simulink library "Generator_Lib"  (R2019a)
settings: Solver=VariableStepAuto  StartTime=0.0  StopTime=10.0  RelTol=1e-3
undefined symbols (not defined in the file): block_angle, D1, Delta, DiscIntNeverNeededParam, fao, Ts
libraries: powerlib x56, powerlib_extras x9, simulink x8, sps_avr x2, powerlib_meascontrol x2
(part 1 of 2)
settings Model: Creator=smiller  LastModifiedBy=smiller

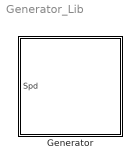
== system Generator_Lib ==
  Generator : Subsystem  VariantControlMode=Label  Variant=on  LabelModeActiveChoice=VSCF_DC_Link  mask{GenType=VSCF DC Link, GenTypeDCLink=Ideal}
      mask prompts: GenType "Generator Type"; GenTypeDCLink "Generator Type, DC Link"
      mask init:
      | set_param(gcb,'LabelModeActiveChoice',strrep(get_param(gcb,'GenType'),' ','_'));
      | set_param([gcb '/VSCF DC Link'],'GenTypeDCLink',get_param(gcb,'GenTypeDCLink'));
      settings: AttributesFormatString=%<BlockChoice>
      mask TypeOptions GenType: Ideal | Integrated Drive | VSCF Cycloconverter | VSCF DC Link
      mask TypeOptions GenTypeDCLink: Ideal | Sync Mach
      mask Display:
      | blk=find_system(gcbh, 'SearchDepth', 1,'FollowLinks','on','LookUnderMasks','all', 'Parent', gcb,'VariantObject', get_param(gcb,'activevariant'));
      | eval(get_param(blk, 'MaskDisplay'));

== system Generator_Lib/Generator ==
  Spd : Inport
  Ideal : Subsystem  VariantControl=Ideal
      mask Display: image(imread('Gen_Ideal_IMAGE.jpg'));
  Integrated Drive : Subsystem  VariantControl=Integrated_Drive
      mask Display: image(imread('Gen_IDG_IMAGE.jpg'))
  VSCF Cycloconverter : Subsystem  VariantControl=VSCF_Cycloconverter
      mask Display: image(imread('Gen_VSCF_Cycloconverter_IMAGE.jpg'))
  VSCF DC Link : Subsystem  VariantControl=VSCF_DC_Link  mask{GenTypeDCLink=Ideal}
      mask prompts: GenTypeDCLink "Generator Type"
      mask init:
      | set_param([gcb '/DC Link Gen'],'GenTypeDCLink',get_param(gcb,'GenTypeDCLink'));
      mask TypeOptions GenTypeDCLink: Ideal | Sync Mach
      mask Display: image('Gen_VSCF_DCLink_IMAGE.jpg');
  A : PMIOPort  Side=Right
  B : PMIOPort  Port=2  Side=Right
  C : PMIOPort  Port=3  Side=Right

== system Generator_Lib/Generator/Ideal ==
  Spd : Inport
  Parasitic Resistive Load : powerlib/Elements/Three-Phase Series RLC Load  LConnTagsString=A|B|C  Configuration=Y (grounded)  NominalVoltage=200  Vabc=[1e3 1e3 1e3]  Vabcp=[1e3 1e3 1e3]  NominalFrequency=400  UnbalancedPower=off  ActivePower=5000  InductivePower=0  CapacitivePower=0  Pabc=[10e3 9e3 11e3]  QLabc=[100 90 110]  QCabc=[100 90 110]  Pabcp=[10e3 9e3 11e3]  QLabcp=[100 90 110]  QCabcp=[100 90 110]  Measurements=None  LoadType=constant Z
      settings: SourceProductName=Simscape Electrical
  Sensing : Subsystem
      mask Display: disp('S')
  Terminator : Terminator
  Three-Phase V-I Measurement4 : powerlib/Measurements/Three-Phase V-I Measurement  VoltageMeasurement=phase-to-ground  SetLabelV=on  LabelV=Vabc_Gen1Only  Vpu=off  VpuLL=off  CurrentMeasurement=yes  SetLabelI=on  LabelI=Iabc_Gen1Only  Ipu=off  Pbase=100e6  Vbase=500e3  OutputType=Magnitude  PhasorSimulation=on  PSBequivalent=0
      settings: SourceProductName=Simscape Electrical
  Three-Phase Source : powerlib/Electrical Sources/Three-Phase Source  InternalConnection=Yg  VoltagePhases=off  Voltage=200  PhaseAngle=0  Voltage_phases=[25e3 25e3 25e3]/sqrt(3)  PhaseAngles_phases=[0 -120 +120]  Frequency=400  NonIdealSource=on  SpecifyImpedance=off  Resistance=0.1*0  Inductance=0.01*0  ShortCircuitLevel=0.1  BaseVoltage=200  XRratio=7  BusType=swing  Pref=0  Qref=0  Prefabc=[10e3, 10e3, 10e3]  Qrefabc=[0, 0, 0]  Qmin=-inf  Qmax=inf
      settings: SourceProductName=Simscape Electrical
  Vab : Subsystem
  rpm2 radps : Gain  Gain=pi/30
  A : PMIOPort  Side=Right
  B : PMIOPort  Port=2  Side=Right
  C : PMIOPort  Port=3  Side=Right
  wires:
  rpm2 radps/1 -> Terminator/1
  Spd/1 -> rpm2 radps/1
  connections:
  Three-Phase V-I Measurement4/LConn3 -- Three-Phase Source/RConn3
  Three-Phase V-I Measurement4/LConn2 -- Three-Phase Source/RConn2
  Three-Phase V-I Measurement4/LConn1 -- Three-Phase Source/RConn1
  A/RConn1 -- Parasitic Resistive Load/LConn1 -- Three-Phase V-I Measurement4/RConn1 -- Vab/RConn1
  C/RConn1 -- Three-Phase V-I Measurement4/RConn3 -- Parasitic Resistive Load/LConn3
  B/RConn1 -- Parasitic Resistive Load/LConn2 -- Three-Phase V-I Measurement4/RConn2 -- Vab/RConn2

== system Generator_Lib/Generator/Integrated Drive ==
  Spd : Inport
  Bus Selector2 : BusSelector  OutputSignals=Rotor speed wm (rad/s)
  Displays : Subsystem
  Generator Control Unit (GCU) : Subsystem
      mask Display: %image(imread('power_aircraft_distribution_GCU.jpg','jpg'))
  Generator Control Breaker (GCB) : Subsystem
  IDG : Subsystem
  Parasitic Resistive Load : powerlib/Elements/Three-Phase Series RLC Load  LConnTagsString=A|B|C  Configuration=Y (grounded)  NominalVoltage=200  Vabc=[1e3 1e3 1e3]  Vabcp=[1e3 1e3 1e3]  NominalFrequency=400  UnbalancedPower=off  ActivePower=5000  InductivePower=0  CapacitivePower=0  Pabc=[10e3 9e3 11e3]  QLabc=[100 90 110]  QCabc=[100 90 110]  Pabcp=[10e3 9e3 11e3]  QLabcp=[100 90 110]  QCabcp=[100 90 110]  Measurements=None  LoadType=constant Z
      settings: SourceProductName=Simscape Electrical
  Sensing : Subsystem
      mask Display: disp('S')
  Simplified Synchronous Machine SI Units : powerlib/Machines/Simplified Synchronous Machine SI Units  ConnectionType=3-wire Y  MechanicalLoad=Speed w  MeasurementBus=off  NominalParameters=[50e3 200 400]  Mechanical=[0.02 0 2]  InternalRL="[0.0204  0.08104e-3]"  InitialConditions=[-99 1.73677 24.5109 24.5109 24.5109 -1.98949 -121.989 118.011]  Units=1  LoadFlowParameters=[1 0 0 0 0]  TsPowergui=0  TsBlock=-1  BusType=swing  Pref=0  Qref=0  Qmin=-inf  Qmax=+inf  PLF=0  QLF=0
      settings: SourceProductName=Simscape Electrical  SourceProductBaseCode=PS
  Vab : Subsystem
  A : PMIOPort  Side=Right
  B : PMIOPort  Port=2  Side=Right
  C : PMIOPort  Port=3  Side=Right
  wires:
  IDG/1(Dr) -> Simplified Synchronous Machine SI Units/1
  Spd/1 -> IDG/1(Tur)
  Generator Control Breaker (GCB)/2(Iabc) -> Generator Control Unit (GCU)/1(Iabc)
  Generator Control Unit (GCU)/1(V Field) -> Simplified Synchronous Machine SI Units/2  "Field"
  Bus Selector2/1 -> Displays/1(w), Generator Control Unit (GCU)/3(PMG), Generator Control Breaker (GCB)/1(GLC)  "<Rotor speed wm (rad/s)>"
  Generator Control Breaker (GCB)/1(Vabc) -> Generator Control Unit (GCU)/2(Vabc)
  Simplified Synchronous Machine SI Units/1 -> Bus Selector2/1, Sensing/1(In1)
  connections:
  Simplified Synchronous Machine SI Units/RConn1 -- Generator Control Breaker (GCB)/LConn1 -- Parasitic Resistive Load/LConn1
  Simplified Synchronous Machine SI Units/RConn2 -- Generator Control Breaker (GCB)/LConn2 -- Parasitic Resistive Load/LConn2
  Simplified Synchronous Machine SI Units/RConn3 -- Parasitic Resistive Load/LConn3 -- Generator Control Breaker (GCB)/LConn3
  Generator Control Breaker (GCB)/RConn2 -- Vab/RConn2 -- B/RConn1
  C/RConn1 -- Generator Control Breaker (GCB)/RConn3
  Generator Control Breaker (GCB)/RConn1 -- Vab/RConn1 -- A/RConn1

== system Generator_Lib/Generator/VSCF Cycloconverter ==
  Spd : Inport
  AC Generator Cycloconverter : Subsystem
  Constant : Constant  Value=[0 0 0]
  Generator Control Breaker (GCB) : Subsystem
  Terminator : Terminator
  Terminator1 : Terminator
  Vab : Subsystem
  A : PMIOPort  Side=Right
  B : PMIOPort  Port=2  Side=Right
  C : PMIOPort  Port=3  Side=Right
  tag scope: Gen1Bus=global
  wires:
  Generator Control Breaker (GCB)/2(Iabc) -> Terminator1/1
  Generator Control Breaker (GCB)/1(Vabc) -> Terminator/1
  Constant/1 -> [Gen1Bus]
  Spd/1 -> Generator Control Breaker (GCB)/1(GLC), AC Generator Cycloconverter/1(rpm)
  connections:
  AC Generator Cycloconverter/RConn1 -- Generator Control Breaker (GCB)/LConn1
  AC Generator Cycloconverter/RConn2 -- Generator Control Breaker (GCB)/LConn2
  AC Generator Cycloconverter/RConn3 -- Generator Control Breaker (GCB)/LConn3
  B/RConn1 -- Generator Control Breaker (GCB)/RConn2 -- Vab/RConn2
  C/RConn1 -- Generator Control Breaker (GCB)/RConn3
  A/RConn1 -- Generator Control Breaker (GCB)/RConn1 -- Vab/RConn1

== system Generator_Lib/Generator/VSCF DC Link ==
  note: AC-DC-AC PWM Converter
  Spd : Inport
  Constant : Constant  Value=[0 0 0]
  DC Link Gen : Subsystem  VariantControlMode=Label  Variant=on  LabelModeActiveChoice=Ideal  mask{GenTypeDCLink=Ideal}
      mask prompts: GenTypeDCLink "Generator Type, DC Link"
      mask init:
      | set_param(gcb,'LabelModeActiveChoice',strrep(get_param(gcb,'GenTypeDCLink'),' ','_'));
      settings: AttributesFormatString=%<BlockChoice>
      mask TypeOptions GenTypeDCLink: Ideal | Sync Mach
  LC Filter : Subsystem
  Meas : powerlib/Measurements/Three-Phase V-I Measurement  VoltageMeasurement=phase-to-ground  SetLabelV=off  LabelV=V1  Vpu=on  VpuLL=off  CurrentMeasurement=no  SetLabelI=off  LabelI=I1  Ipu=off  Pbase=1e3  Vbase=200  OutputType=Magnitude  PhasorSimulation=off  PSBequivalent=0
      settings: SourceProductName=Simscape Electrical
  Rect and Inv : Subsystem
  Regulator : Subsystem
  Subsystem2 : Subsystem
      mask Display: disp('S')
  Subsystem4 : Subsystem
      mask Display: disp('S')
  Subsystem5 : Subsystem
      mask Display: disp('S')
  Transformer : powerlib/Elements/Three-Phase Transformer (Two Windings)  Winding1Connection=Yg  Winding2Connection=Delta (D1)  CoreType=Three single-phase transformers  SetSaturation=off  Hysteresis=off  DataFile='hysteresis'  SetInitialFlux=off  Measurements=None  UNITS=pu  NominalPower=[ 50e3 , 800 ]  Winding1=[ 200 , 0.004 , 0.02 ]  Winding2=[ 600 , 0.004 , 0.02 ]  Rm=200  Lm=200  L0=0.5  Saturation="[ 0,0  ;  0.005,1.2  ;  1.0,1.4 ]"  InitialFluxes=[ 0.8 , -0.8 , 0.7 ]  BreakLoop=off  DiscreteSolver=Trapezoidal iterative  DataType=off  TransfoNumber=0
      settings: SourceProductName=Simscape Electrical
  "Vref (pu) " : Constant
  A : PMIOPort  Side=Right
  B : PMIOPort  Port=2  Side=Right
  C : PMIOPort  Port=3  Side=Right
  tag scope: Gen1Bus=global
  wires:
  Constant/1 -> [Gen1Bus]
  Spd/1 -> DC Link Gen/1(rpm)
  Regulator/1(g) -> Rect and Inv/1(g)
  Meas/1 -> Regulator/2(Vabc (pu))
  "Vref (pu) "/1 -> Regulator/1(Vref (pu))
  connections:
  Rect and Inv/RConn3 -- LC Filter/LConn3
  Transformer/RConn3 -- Rect and Inv/LConn3
  Rect and Inv/LConn2 -- Transformer/RConn2
  DC Link Gen/RConn3 -- Transformer/LConn3
  Transformer/RConn1 -- Rect and Inv/LConn1
  Meas/LConn3 -- LC Filter/RConn3
  Meas/RConn3 -- C/RConn1
  Meas/LConn2 -- LC Filter/RConn2
  DC Link Gen/RConn2 -- Transformer/LConn2
  Meas/LConn1 -- LC Filter/RConn1
  B/RConn1 -- Meas/RConn2
  Rect and Inv/RConn1 -- Subsystem5/LConn1 -- LC Filter/LConn1
  Subsystem5/LConn2 -- Rect and Inv/RConn2 -- LC Filter/LConn2
  Subsystem2/LConn1 -- DC Link Gen/RConn1 -- Transformer/LConn1
  Meas/RConn1 -- A/RConn1 -- Subsystem4/LConn1

== system Generator_Lib/Generator/Ideal/Sensing ==
  Constant : Constant  Value=[1 1]*12000  SampleTime=-1
  Constant1 : Constant  Value=202  SampleTime=-1
  Mux : Mux  Inputs=3
  rpm2pu1 : Gain  Gain=2*pi/60
  tag scope: Gen1Data=global
  wires:
  Constant/1 -> rpm2pu1/1  "Spd"
  Mux/1 -> [Gen1Data]
  rpm2pu1/1 -> Mux/1
  Constant1/1 -> Mux/2
  [Pwr_Gen1_Only] -> Mux/3

== system Generator_Lib/Generator/Ideal/Vab ==
  Voltage Measurement : powerlib/Measurements/Voltage Measurement  PhasorSimulation=off  OutputType=Magnitude  PSBequivalent=0
      settings: SourceProductName=Simscape Electrical
  + : PMIOPort  Side=Right
  - : PMIOPort  Port=2  Side=Right
  tag scope: Gen1_Vab=global
  wires:
  Voltage Measurement/1 -> [Gen1_Vab]
  connections:
  Voltage Measurement/LConn2 -- -/RConn1
  Voltage Measurement/LConn1 -- +/RConn1

== system Generator_Lib/Generator/Integrated Drive/Displays ==
  w : Inport
  Frequency (Hz) : Display
      settings: Decimation=100  SampleTime=1e-2
  Gain : Gain  Gain=30/pi
  Gain3 : Gain  Gain=1/30
  Rate Transition : RateTransition  OutPortSampleTimeOpt=Inherit  OutPortSampleTime=Ts
  Rate Transition1 : RateTransition  OutPortSampleTimeOpt=Inherit  OutPortSampleTime=Ts
  Speed (RPM) : Display
      settings: Decimation=100  SampleTime=1e-2
  wires:
  Rate Transition1/1 -> Frequency (Hz)/1
  Gain/1 -> Gain3/1, Rate Transition/1
  Gain3/1 -> Rate Transition1/1
  Rate Transition/1 -> Speed (RPM)/1
  w/1 -> Gain/1

== system Generator_Lib/Generator/Integrated Drive/Generator Control Unit (GCU) ==
  Iabc : Inport
  Vabc : Inport  Port=2
  PMG : Inport  Port=3
  Demux : Demux  Outputs=3
  Excitation System : sps_avr/Excitation System  tr=20e-3  reg=[ 300, 0.001 ]  exc=[ 1, 0 ]  tgr=[ 0, 0 ]  damp=[ 0.001, 0.1 ]  sat=[ 0, 0 ]  lim=[ -2, 2, 0 ]  v0=[1 1*203.1/200]
      settings: SourceProductName=Simscape Electrical  SourceProductBaseCode=PS
  Integrator : Integrator
  PU_SI : Gain  Gain=200
  SI_PU : Gain  Gain=1/(200*sqrt(2))
  Terminator1 : Terminator
  Terminator2 : Terminator
  Vref : Constant
  abc to dq0 : powerlib_meascontrol/Transformations/abc to dq0  Alignment=90 degrees behind phase A axis
      settings: SourceProductName=Simscape Electrical
  threshold3 : Constant  Value=0
  V Field : Outport
  tag scope: Gen1_Vfield=global
  wires:
  Demux/3 -> Terminator2/1
  Iabc/1 -> Terminator1/1
  threshold3/1 -> Excitation System/4
  Vref/1 -> Excitation System/1
  PU_SI/1 -> [Gen1_Vfield], V Field/1
  Excitation System/1 -> PU_SI/1
  SI_PU/1 -> abc to dq0/1
  Demux/2 -> Excitation System/3
  Demux/1 -> Excitation System/2
  abc to dq0/1 -> Demux/1
  Integrator/1 -> abc to dq0/2
  PMG/1 -> Integrator/1
  Vabc/1 -> SI_PU/1

== system Generator_Lib/Generator/Integrated Drive/Generator Control Breaker (GCB) ==
  GLC : Inport
  Close switch : Subsystem
  Complex to Real-Imag : ComplexToRealImag  Output=Real
  Complex to Real-Imag1 : ComplexToRealImag  Output=Real
  Contactor : Subsystem
  Memory : Memory
  P.O.R  and CTA : powerlib/Measurements/Three-Phase V-I Measurement  VoltageMeasurement=phase-to-phase  SetLabelV=off  LabelV=Vabc_Gen1  Vpu=off  VpuLL=off  CurrentMeasurement=yes  SetLabelI=off  LabelI=Iabc_Gen1  Ipu=off  Pbase=100e6  Vbase=500e3  OutputType=Complex  PhasorSimulation=off  PSBequivalent=0
      settings: SourceProductName=Simscape Electrical
  in_a : PMIOPort  Side=Left
  in_b : PMIOPort  Port=2  Side=Left
  in_c : PMIOPort  Port=3  Side=Left
  out_a : PMIOPort  Port=4  Side=Right
  out_b : PMIOPort  Port=5  Side=Right
  out_c : PMIOPort  Port=6  Side=Right
  Vabc : Outport
  Iabc : Outport  Port=2
  wires:
  GLC/1 -> Memory/1
  P.O.R  and CTA/1 -> Complex to Real-Imag/1
  P.O.R  and CTA/2 -> Complex to Real-Imag1/1
  Complex to Real-Imag/1 -> Vabc/1
  Complex to Real-Imag1/1 -> Iabc/1
  Memory/1 -> Close switch/1(In1)
  Close switch/1(Out1) -> Contactor/1(com)
  connections:
  out_b/RConn1 -- Contactor/RConn2
  Contactor/LConn1 -- P.O.R  and CTA/RConn1
  P.O.R  and CTA/LConn1 -- in_a/RConn1
  in_b/RConn1 -- P.O.R  and CTA/LConn2
  P.O.R  and CTA/LConn3 -- in_c/RConn1
  Contactor/LConn3 -- P.O.R  and CTA/RConn3
  P.O.R  and CTA/RConn2 -- Contactor/LConn2
  Contactor/RConn1 -- out_a/RConn1
  Contactor/RConn3 -- out_c/RConn1

== system Generator_Lib/Generator/Integrated Drive/IDG ==
  Tur : Inport
  Constant : Constant  Value=12000*pi/30
  Terminator : Terminator
  rpm2 radps : Gain  Gain=pi/30
  Dr : Outport
  wires:
  Constant/1 -> Dr/1
  Tur/1 -> rpm2 radps/1
  rpm2 radps/1 -> Terminator/1

== system Generator_Lib/Generator/Integrated Drive/Sensing ==
  In1 : Inport
  Data : Subsystem
  Mux : Mux  Inputs=3
  tag scope: Gen1Data=global
  wires:
  Data/3(Pe) -> Mux/3
  Data/2(Vf) -> Mux/2
  Data/1(w) -> Mux/1
  In1/1 -> Data/1(B)
  Mux/1 -> [Gen1Data]

== system Generator_Lib/Generator/Integrated Drive/Vab ==
  Voltage Measurement : powerlib/Measurements/Voltage Measurement  PhasorSimulation=off  OutputType=Magnitude  PSBequivalent=0
      settings: SourceProductName=Simscape Electrical
  + : PMIOPort  Side=Right
  - : PMIOPort  Port=2  Side=Right
  tag scope: Gen1_Vab=global
  wires:
  Voltage Measurement/1 -> [Gen1_Vab]
  connections:
  Voltage Measurement/LConn1 -- +/RConn1
  Voltage Measurement/LConn2 -- -/RConn1

== system Generator_Lib/Generator/VSCF Cycloconverter/AC Generator Cycloconverter ==
  rpm : Inport
  Cycloconverter control (Vsync) : Subsystem
  Ground1 : powerlib/Elements/Ground  LConnTagsString=a
      settings: SourceProductName=Simscape Electrical
  Ideal Source : Subsystem
  Load Measurements : powerlib/Measurements/Three-Phase V-I Measurement  VoltageMeasurement=phase-to-ground  SetLabelV=on  LabelV=Vload  Vpu=off  VpuLL=off  CurrentMeasurement=yes  SetLabelI=on  LabelI=Iload  Ipu=off  Pbase=100e6  Vbase=500e3  OutputType=Complex  PhasorSimulation=off  PSBequivalent=0
      settings: SourceProductName=Simscape Electrical
  Phase A Cycloconverter : Subsystem
  Phase B Cycloconverter : Subsystem
  Phase C Cycloconverter : Subsystem
  Source Measurements : powerlib/Measurements/Three-Phase V-I Measurement  VoltageMeasurement=phase-to-ground  SetLabelV=on  LabelV=Vsource  Vpu=off  VpuLL=off  CurrentMeasurement=yes  SetLabelI=on  LabelI=Isource  Ipu=off  Pbase=100e6  Vbase=500e3  OutputType=Complex  PhasorSimulation=off  PSBequivalent=0
      settings: SourceProductName=Simscape Electrical
  Three-Phase Transformer (Two Windings)1 : powerlib/Elements/Three-Phase Transformer (Two Windings)  Winding1Connection=Delta (D1)  Winding2Connection=Delta (D1)  CoreType=Three single-phase transformers  SetSaturation=off  Hysteresis=off  DataFile='hysteresis'  SetInitialFlux=off  Measurements=None  UNITS=pu  NominalPower=[3e6 3000]  Winding1=[200 0 0]  Winding2=[200/sqrt(3) 1e-8 0]  Rm=Inf  Lm=Inf  L0=0.5  Saturation=[ 0,0 ; 0.0024,1.2 ; 1.0,1.52 ]  InitialFluxes=[ 0.8 , -0.8 , 0.7 ]  BreakLoop=off  DiscreteSolver=Trapezoidal iterative  DataType=off  TransfoNumber=1
      settings: SourceProductName=Simscape Electrical
  Three-Phase Transformer (Two Windings)2 : powerlib/Elements/Three-Phase Transformer (Two Windings)  Winding1Connection=Delta (D1)  Winding2Connection=Delta (D1)  CoreType=Three single-phase transformers  SetSaturation=off  Hysteresis=off  DataFile='hysteresis'  SetInitialFlux=off  Measurements=None  UNITS=pu  NominalPower=[3e6 3000]  Winding1=[200 0 0]  Winding2=[200/sqrt(3) 1e-8 0]  Rm=Inf  Lm=Inf  L0=0.5  Saturation=[ 0,0 ; 0.0024,1.2 ; 1.0,1.52 ]  InitialFluxes=[ 0.8 , -0.8 , 0.7 ]  BreakLoop=off  DiscreteSolver=Trapezoidal iterative  DataType=off  TransfoNumber=1
      settings: SourceProductName=Simscape Electrical
  Three-Phase Transformer (Two Windings)3 : powerlib/Elements/Three-Phase Transformer (Two Windings)  Winding1Connection=Delta (D1)  Winding2Connection=Delta (D1)  CoreType=Three single-phase transformers  SetSaturation=off  Hysteresis=off  DataFile='hysteresis'  SetInitialFlux=off  Measurements=None  UNITS=pu  NominalPower=[3e6 3000]  Winding1=[200 0 0]  Winding2=[200/sqrt(3) 1e-8 0]  Rm=Inf  Lm=Inf  L0=0.5  Saturation=[ 0,0 ; 0.0024,1.2 ; 1.0,1.52 ]  InitialFluxes=[ 0.8 , -0.8 , 0.7 ]  BreakLoop=off  DiscreteSolver=Trapezoidal iterative  DataType=off  TransfoNumber=1
      settings: SourceProductName=Simscape Electrical
  Vsync Measurement : powerlib/Measurements/Three-Phase V-I Measurement  VoltageMeasurement=phase-to-phase  SetLabelV=on  LabelV=Vsync  Vpu=off  VpuLL=off  CurrentMeasurement=no  SetLabelI=off  LabelI=Iabc  Ipu=off  Pbase=100e6  Vbase=500e3  OutputType=Complex  PhasorSimulation=off  PSBequivalent=0
      settings: SourceProductName=Simscape Electrical
  A : PMIOPort  Side=Right
  B : PMIOPort  Port=2  Side=Right
  C : PMIOPort  Port=3  Side=Right
  wires:
  rpm/1 -> Ideal Source/1(rpm)
  connections:
  Three-Phase Transformer (Two Windings)1/RConn3 -- Phase B Cycloconverter/LConn3
  Ideal Source/RConn3 -- Source Measurements/LConn3
  Load Measurements/RConn2 -- B/RConn1
  Ideal Source/RConn1 -- Source Measurements/LConn1
  Three-Phase Transformer (Two Windings)3/RConn2 -- Vsync Measurement/LConn2
  Source Measurements/LConn2 -- Ideal Source/RConn2
  Phase C Cycloconverter/LConn3 -- Three-Phase Transformer (Two Windings)2/RConn3
  Load Measurements/RConn3 -- C/RConn1
  Vsync Measurement/RConn3 -- Phase A Cycloconverter/LConn3
  Phase C Cycloconverter/RConn1 -- Load Measurements/LConn3
  Three-Phase Transformer (Two Windings)1/LConn2 -- Three-Phase Transformer (Two Windings)2/LConn2 -- Three-Phase Transformer (Two Windings)3/LConn2 -- Source Measurements/RConn2
  Three-Phase Transformer (Two Windings)1/LConn1 -- Three-Phase Transformer (Two Windings)2/LConn1 -- Three-Phase Transformer (Two Windings)3/LConn1 -- Source Measurements/RConn1
  Phase A Cycloconverter/RConn1 -- Load Measurements/LConn1
  Phase C Cycloconverter/LConn1 -- Three-Phase Transformer (Two Windings)2/RConn1
  Three-Phase Transformer (Two Windings)3/RConn1 -- Vsync Measurement/LConn1
  Phase B Cycloconverter/LConn2 -- Three-Phase Transformer (Two Windings)1/RConn2
  Phase B Cycloconverter/LConn1 -- Three-Phase Transformer (Two Windings)1/RConn1
  Vsync Measurement/RConn1 -- Phase A Cycloconverter/LConn1
  Phase B Cycloconverter/RConn1 -- Load Measurements/LConn2
  Three-Phase Transformer (Two Windings)1/LConn3 -- Source Measurements/RConn3 -- Three-Phase Transformer (Two Windings)3/LConn3 -- Three-Phase Transformer (Two Windings)2/LConn3
  Three-Phase Transformer (Two Windings)2/RConn2 -- Phase C Cycloconverter/LConn2
  Ground1/LConn1 -- Phase B Cycloconverter/RConn2 -- Phase A Cycloconverter/RConn2 -- Phase C Cycloconverter/RConn2
  Three-Phase Transformer (Two Windings)3/RConn3 -- Vsync Measurement/LConn3
  Phase A Cycloconverter/LConn2 -- Vsync Measurement/RConn2
  Load Measurements/RConn1 -- A/RConn1

== system Generator_Lib/Generator/VSCF Cycloconverter/Generator Control Breaker (GCB) ==
  GLC : Inport
  Close switch : Subsystem
  Complex to Real-Imag : ComplexToRealImag  Output=Real
  Complex to Real-Imag1 : ComplexToRealImag  Output=Real
  Contactor : Subsystem
  Memory : Memory
  P.O.R  and CTA : powerlib/Measurements/Three-Phase V-I Measurement  VoltageMeasurement=phase-to-phase  SetLabelV=off  LabelV=Vabc_Gen1  Vpu=off  VpuLL=off  CurrentMeasurement=yes  SetLabelI=off  LabelI=Iabc_Gen1  Ipu=off  Pbase=100e6  Vbase=500e3  OutputType=Complex  PhasorSimulation=off  PSBequivalent=0
      settings: SourceProductName=Simscape Electrical
  in_a : PMIOPort  Side=Left
  in_b : PMIOPort  Port=2  Side=Left
  in_c : PMIOPort  Port=3  Side=Left
  out_a : PMIOPort  Port=4  Side=Right
  out_b : PMIOPort  Port=5  Side=Right
  out_c : PMIOPort  Port=6  Side=Right
  Vabc : Outport
  Iabc : Outport  Port=2
  wires:
  GLC/1 -> Memory/1
  P.O.R  and CTA/1 -> Complex to Real-Imag/1
  P.O.R  and CTA/2 -> Complex to Real-Imag1/1
  Complex to Real-Imag/1 -> Vabc/1
  Complex to Real-Imag1/1 -> Iabc/1
  Memory/1 -> Close switch/1(In1)
  Close switch/1(Out1) -> Contactor/1(com)
  connections:
  out_b/RConn1 -- Contactor/RConn2
  Contactor/LConn1 -- P.O.R  and CTA/RConn1
  P.O.R  and CTA/LConn1 -- in_a/RConn1
  in_b/RConn1 -- P.O.R  and CTA/LConn2
  P.O.R  and CTA/LConn3 -- in_c/RConn1
  Contactor/LConn3 -- P.O.R  and CTA/RConn3
  P.O.R  and CTA/RConn2 -- Contactor/LConn2
  Contactor/RConn1 -- out_a/RConn1
  Contactor/RConn3 -- out_c/RConn1

== system Generator_Lib/Generator/VSCF Cycloconverter/Vab ==
  Voltage Measurement : powerlib/Measurements/Voltage Measurement  PhasorSimulation=off  OutputType=Magnitude  PSBequivalent=0
      settings: SourceProductName=Simscape Electrical
  + : PMIOPort  Side=Right
  - : PMIOPort  Port=2  Side=Right
  tag scope: Gen1_Vab=global
  wires:
  Voltage Measurement/1 -> [Gen1_Vab]
  connections:
  Voltage Measurement/LConn1 -- +/RConn1
  Voltage Measurement/LConn2 -- -/RConn1

== system Generator_Lib/Generator/VSCF DC Link/DC Link Gen ==
  rpm : Inport
  Ideal : Subsystem  VariantControl=Ideal
      mask Display: image(imread('Gen_Ideal_Var_IMAGE.jpg'));
  Sync Mach : Subsystem  VariantControl=Sync_Mach
      mask Display: image(imread('Gen_Sync_Machine_IMAGE.jpg'));
  A : PMIOPort  Side=Right
  B : PMIOPort  Port=2  Side=Right
  C : PMIOPort  Port=3  Side=Right

== system Generator_Lib/Generator/VSCF DC Link/LC Filter ==
  Capacitor : powerlib/Elements/Three-Phase Series RLC Load  LConnTagsString=A|B|C  Configuration=Y (grounded)  NominalVoltage=200  Vabc=[1e3 1e3 1e3]  Vabcp=[1e3 1e3 1e3]  NominalFrequency=400  UnbalancedPower=off  ActivePower=0  InductivePower=0  CapacitivePower=3e3  Pabc=[10e3 9e3 11e3]  QLabc=[100 90 110]  QCabc=[100 90 110]  Pabcp=[10e3 9e3 11e3]  QLabcp=[100 90 110]  QCabcp=[100 90 110]  Measurements=None  LoadType=constant Z
      settings: SourceProductName=Simscape Electrical
  Inductor : powerlib/Elements/Three-Phase Series RLC Branch  LConnTagsString=A|B|C  RConnTagsString=A|B|C  BranchType=L  Resistance=0  Inductance=2e-3*0.43  Capacitance=inf  Measurements=None
      settings: SourceProductName=Simscape Electrical
  A : PMIOPort  Side=Left
  B : PMIOPort  Port=2  Side=Left
  C : PMIOPort  Port=3  Side=Left
  "A " : PMIOPort  Port=4  Side=Right
  "B " : PMIOPort  Port=5  Side=Right
  "C " : PMIOPort  Port=6  Side=Right
  connections:
  "C "/RConn1 -- Capacitor/LConn3 -- Inductor/RConn3
  Capacitor/LConn2 -- "B "/RConn1 -- Inductor/RConn2
  Capacitor/LConn1 -- "A "/RConn1 -- Inductor/RConn1
  C/RConn1 -- Inductor/LConn3
  A/RConn1 -- Inductor/LConn1
  B/RConn1 -- Inductor/LConn2

== system Generator_Lib/Generator/VSCF DC Link/Rect and Inv ==
  g : Inport
  C1 : powerlib/Elements/Parallel RLC Branch  LConnTagsString=a  RConnTagsString=__new0  BranchType=C  Resistance=inf  Inductance=inf  SetiL0=off  InitialCurrent=0  Capacitance=5000e-06  Setx0=on  InitialVoltage=797  Measurements=None
      settings: SourceProductName=Simscape Electrical
  L1 : powerlib/Elements/Series RLC Branch  LConnTagsString=__new0  RConnTagsString=__new0  BranchType=L  Resistance=1.0  Inductance=200e-6  SetiL0=off  InitialCurrent=0  Capacitance=1.0  Setx0=off  InitialVoltage=0  Measurements=None
      settings: SourceProductName=Simscape Electrical
  PWM IGBT Inverter : powerlib/Power Electronics/Universal Bridge  Arms=3  SnubberResistance=5000  SnubberCapacitance=inf  Device=IGBT / Diodes  Ron=1e-3  Lon=0  ForwardVoltages="[  0.0  0.0  ]"  ForwardVoltage=.8  GTOparameters=[ 1e-6 ,1e-6 ]  IGBTparameters=[ 1e-6 , 2e-6 ]  Measurements=Device currents  Measurements_2=None  converterType=Rectifier
      settings: SourceProductName=Simscape Electrical
  Rectifier : powerlib/Power Electronics/Universal Bridge  Arms=3  SnubberResistance=100  SnubberCapacitance=0.1e-6  Device=Diodes  Ron=1e-3  Lon=0  ForwardVoltages="[  0.8  0.8  ]"  ForwardVoltage=.8  GTOparameters=[ 10e-6 , 20e-6 ]  IGBTparameters=[ 1e-6 , 2e-6 ]  Measurements=Device currents  Measurements_2=None  converterType=Rectifier
      settings: SourceProductName=Simscape Electrical
  Subsystem3 : Subsystem
      mask Display: disp('S')
  Ar : PMIOPort  Side=Left
  Ai : PMIOPort  Port=2  Side=Right
  Br : PMIOPort  Port=3  Side=Left
  Bi : PMIOPort  Port=4  Side=Right
  Cr : PMIOPort  Port=5  Side=Left
  Ci : PMIOPort  Port=6  Side=Right
  wires:
  g/1 -> PWM IGBT Inverter/1
  connections:
  PWM IGBT Inverter/LConn1 -- Ai/RConn1
  PWM IGBT Inverter/LConn2 -- Bi/RConn1
  Rectifier/LConn2 -- Br/RConn1
  Ar/RConn1 -- Rectifier/LConn1
  Cr/RConn1 -- Rectifier/LConn3
  Subsystem3/LConn1 -- PWM IGBT Inverter/RConn1 -- C1/LConn1 -- L1/RConn1
  Subsystem3/RConn1 -- Rectifier/RConn2 -- C1/RConn1 -- PWM IGBT Inverter/RConn2
  Rectifier/RConn1 -- L1/LConn1
  PWM IGBT Inverter/LConn3 -- Ci/RConn1

== system Generator_Lib/Generator/VSCF DC Link/Regulator ==
  Vref (pu) : Inport
  Vabc (pu) : Inport  Port=2
  Discrete PWM Generator : powerlib_extras/Discrete  Control Blocks/Discrete PWM Generator  GeneratorMode="3-arm  bridge (6 pulses)"  Fc=10000  Ts=Ts  Internal=off  mIndex=0.4  Freq=60  Phase=0
      settings: SourceProductName=Simscape Electrical  SourceProductBaseCode=PS
  Unit Delay1 : UnitDelay  SampleTime=Ts  HasFrameUpgradeWarning=on
  Voltage Regulator : Subsystem  mask(Voltage Regulator){Kp=0.4, Ki=500, Ts=Ts}
      mask prompts: Kp "Proportional gain  Kp:"; Ki "Integral gain Ki:"; Ts "Sample time (s) :"
  g : Outport
  wires:
  Unit Delay1/1 -> g/1
  Discrete PWM Generator/1 -> Unit Delay1/1
  Vref (pu)/1 -> Voltage Regulator/1(Vd_ref (pu))
  Vabc (pu)/1 -> Voltage Regulator/2(Vabc (pu))
  Voltage Regulator/1(Vabc_inv) -> Discrete PWM Generator/1

== system Generator_Lib/Generator/VSCF DC Link/Subsystem2 ==
  Ground : powerlib/Elements/Ground  LConnTagsString=a
      settings: SourceProductName=Simscape Electrical
  Vdc1 : powerlib/Measurements/Voltage Measurement  Tag=PoWeRsYsTeMmEaSuReMeNt  PhasorSimulation=off  OutputType=Magnitude  PSBequivalent=0
      settings: SourceProductName=Simscape Electrical
  Conn1 : PMIOPort  Side=Left
  tag scope: Va_Src=global
  wires:
  Vdc1/1 -> [Va_Src]
  connections:
  Ground/LConn1 -- Vdc1/LConn2
  Vdc1/LConn1 -- Conn1/RConn1

== system Generator_Lib/Generator/VSCF DC Link/Subsystem4 ==
  Ground : powerlib/Elements/Ground  LConnTagsString=a
      settings: SourceProductName=Simscape Electrical
  Vdc1 : powerlib/Measurements/Voltage Measurement  Tag=PoWeRsYsTeMmEaSuReMeNt  PhasorSimulation=off  OutputType=Magnitude  PSBequivalent=0
      settings: SourceProductName=Simscape Electrical
  Conn1 : PMIOPort  Side=Left
  tag scope: Va_Load=global
  wires:
  Vdc1/1 -> [Va_Load]
  connections:
  Vdc1/LConn1 -- Conn1/RConn1
  Ground/LConn1 -- Vdc1/LConn2

== system Generator_Lib/Generator/VSCF DC Link/Subsystem5 ==
  Vdc : powerlib/Measurements/Voltage Measurement  Tag=PoWeRsYsTeMmEaSuReMeNt  PhasorSimulation=off  OutputType=Magnitude  PSBequivalent=0
      settings: SourceProductName=Simscape Electrical
  + : PMIOPort  Side=Left
  - : PMIOPort  Port=2  Side=Left
  tag scope: Vab_Inv=global
  wires:
  Vdc/1 -> [Vab_Inv]  "Vdc"
  connections:
  Vdc/LConn1 -- +/RConn1
  -/RConn1 -- Vdc/LConn2

== system Generator_Lib/Generator/Integrated Drive/Generator Control Breaker (GCB)/Close switch ==
  In1 : Inport
  Data Type Conversion : DataTypeConversion
  Rad_Rpm : Gain  Gain=30/pi
  Relay : Relay  OnSwitchValue=9000  OffSwitchValue=8900
  Out1 : Outport
  wires:
  Data Type Conversion/1 -> Out1/1
  Rad_Rpm/1 -> Relay/1
  Relay/1 -> Data Type Conversion/1
  In1/1 -> Rad_Rpm/1

== system Generator_Lib/Generator/Integrated Drive/Generator Control Breaker (GCB)/Contactor ==
  com : Inport
  Three-Phase Breaker : powerlib/Elements/Three-Phase Breaker  InitialState=open  SwitchA=on  SwitchB=on  SwitchC=on  SwitchTimes="[4/60  10/60]"  External=on  BreakerResistance=0.001  SnubberResistance=1e3  SnubberCapacitance=inf  Measurements=None
      settings: SourceProductName=Simscape Electrical
  A : PMIOPort  Side=Left
  a : PMIOPort  Port=2  Side=Right
  B : PMIOPort  Port=3  Side=Left
  b : PMIOPort  Port=4  Side=Right
  C : PMIOPort  Port=5  Side=Left
  c : PMIOPort  Port=6  Side=Right
  wires:
  com/1 -> Three-Phase Breaker/1
  connections:
  a/RConn1 -- Three-Phase Breaker/RConn1
  Three-Phase Breaker/RConn2 -- b/RConn1
  c/RConn1 -- Three-Phase Breaker/RConn3
  A/RConn1 -- Three-Phase Breaker/LConn1
  B/RConn1 -- Three-Phase Breaker/LConn2
  C/RConn1 -- Three-Phase Breaker/LConn3

== system Generator_Lib/Generator/Integrated Drive/Sensing/Data ==
  B : Inport
  Bus Selector : BusSelector  OutputSignals=Rotor speed wm (rad/s),Electrical power Pe (W),Terminal voltage Va (V),Terminal voltage Vb (V),Terminal voltage Vc (V),Stator current is_a (A),Stator current is_b (A),Stator current is_c (A)
  Constant : Constant  Value=12000
  Mux : Mux  Inputs=2
  Mux1 : Mux  Inputs=3
  Mux2 : Mux  Inputs=3
  rpm2pu1 : Gain  Gain=2*pi/60
  w : Outport
  Vf : Outport  Port=2
  Pe : Outport  Port=3
  tag scope: Iabc_Gen1Only=global, Vabc_Gen1Only=global
  wires:
  Bus Selector/8 -> Mux2/3  "<Stator current is_c (A)>"
  Bus Selector/7 -> Mux2/2  "<Stator current is_b (A)>"
  Bus Selector/6 -> Mux2/1  "<Stator current is_a (A)>"
  Mux2/1 -> [Iabc_Gen1Only]
  Mux1/1 -> [Vabc_Gen1Only]
  Bus Selector/5 -> Mux1/3  "<Terminal voltage Vc (V)>"
  Bus Selector/4 -> Mux1/2  "<Terminal voltage Vb (V)>"
  Bus Selector/3 -> Mux1/1  "<Terminal voltage Va (V)>"
  Mux/1 -> w/1
  Constant/1 -> rpm2pu1/1  "Spd"
  rpm2pu1/1 -> Mux/2
  Bus Selector/1 -> Mux/1  "<Rotor speed wm (rad/s)>"
  Bus Selector/2 -> Pe/1  "<Electrical power Pe (W)>"
  B/1 -> Bus Selector/1
  [Gen1_Vfield] -> Vf/1

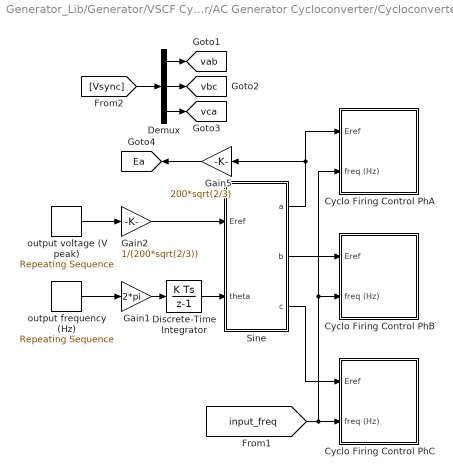
== system Generator_Lib/Generator/VSCF Cycloconverter/AC Generator Cycloconverter/Cycloconverter control (Vsync) ==
  Cyclo Firing Control PhA : Subsystem
  Cyclo Firing Control PhB : Subsystem
  Cyclo Firing Control PhC : Subsystem
  Demux : Demux  Outputs=3
  Discrete-Time Integrator : DiscreteIntegrator  SampleTime=Ts  ICPrevOutput=DiscIntNeverNeededParam  ICPrevScaledInput=DiscIntNeverNeededParam
  Gain1 : Gain  Gain=2*pi
  Gain2 : Gain  Gain=1/(200*sqrt(2/3))
  Gain5 : Gain  Gain=200*sqrt(2/3)
  Sine : Subsystem
  output frequency (Hz) : simulink/Sources/Repeating Sequence  rep_seq_t=[0 10]  rep_seq_y=[1 1]*400
  output voltage (V peak) : simulink/Sources/Repeating Sequence  rep_seq_t=[0 10]  rep_seq_y=[1 1]*200*sqrt(2/3)
  tag scope: Ea=global, vab=global, vbc=global, vca=global
  wires:
  [input_freq] -> Cyclo Firing Control PhB/2(freq (Hz)), Cyclo Firing Control PhA/2(freq (Hz)), Cyclo Firing Control PhC/2(freq (Hz))
  Demux/3 -> [vca]
  Demux/2 -> [vbc]
  Demux/1 -> [vab]
  [Vsync] -> Demux/1
  Gain2/1 -> Sine/1(Eref)
  output voltage (V peak)/1 -> Gain2/1
  Gain5/1 -> [Ea]
  Gain1/1 -> Discrete-Time Integrator/1
  output frequency (Hz)/1 -> Gain1/1
  Sine/3(c) -> Cyclo Firing Control PhC/1(Eref)
  Sine/1(a) -> Gain5/1, Cyclo Firing Control PhA/1(Eref)
  Sine/2(b) -> Cyclo Firing Control PhB/1(Eref)
  Discrete-Time Integrator/1 -> Sine/2(theta)

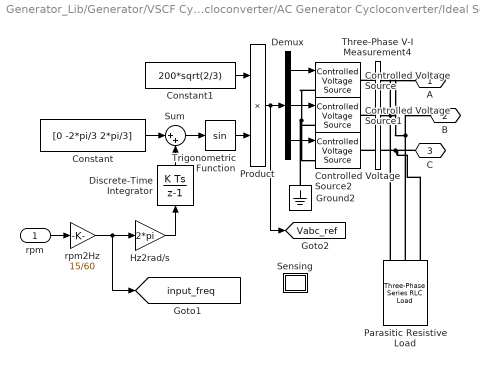
== system Generator_Lib/Generator/VSCF Cycloconverter/AC Generator Cycloconverter/Ideal Source ==
  rpm : Inport
  Constant : Constant  Value=[0 -2*pi/3 2*pi/3]
  Constant1 : Constant  Value=200*sqrt(2/3)
  Controlled Voltage Source : powerlib/Electrical Sources/Controlled Voltage Source  Initialize=off  Source_Type=AC  Amplitude=0  Phase=0  Frequency=0  Measurements=None
      settings: SourceProductName=Simscape Electrical
  Controlled Voltage Source1 : powerlib/Electrical Sources/Controlled Voltage Source  Initialize=off  Source_Type=AC  Amplitude=0  Phase=0  Frequency=0  Measurements=None
      settings: SourceProductName=Simscape Electrical
  Controlled Voltage Source2 : powerlib/Electrical Sources/Controlled Voltage Source  Initialize=off  Source_Type=AC  Amplitude=0  Phase=0  Frequency=0  Measurements=None
      settings: SourceProductName=Simscape Electrical
  Demux : Demux  Outputs=3
  Discrete-Time Integrator : DiscreteIntegrator  SampleTime=Ts  ICPrevOutput=DiscIntNeverNeededParam  ICPrevScaledInput=DiscIntNeverNeededParam
  Ground2 : powerlib/Elements/Ground  LConnTagsString=a
      settings: SourceProductName=Simscape Electrical
  Hz2rad/s : Gain  Gain=2*pi
  Parasitic Resistive Load : powerlib/Elements/Three-Phase Series RLC Load  LConnTagsString=A|B|C  Configuration=Y (grounded)  NominalVoltage=200  Vabc=[1e3 1e3 1e3]  Vabcp=[1e3 1e3 1e3]  NominalFrequency=400  UnbalancedPower=off  ActivePower=5000  InductivePower=0  CapacitivePower=0  Pabc=[10e3 9e3 11e3]  QLabc=[100 90 110]  QCabc=[100 90 110]  Pabcp=[10e3 9e3 11e3]  QLabcp=[100 90 110]  QCabcp=[100 90 110]  Measurements=None  LoadType=constant Z
      settings: SourceProductName=Simscape Electrical
  Product : Product
  Sensing : Subsystem
      mask Display: disp('S')
  Sum : Sum  Inputs=|++
  Three-Phase V-I Measurement4 : powerlib/Measurements/Three-Phase V-I Measurement  VoltageMeasurement=phase-to-ground  SetLabelV=on  LabelV=Vabc_Gen1Only  Vpu=off  VpuLL=off  CurrentMeasurement=yes  SetLabelI=on  LabelI=Iabc_Gen1Only  Ipu=off  Pbase=100e6  Vbase=500e3  OutputType=Magnitude  PhasorSimulation=on  PSBequivalent=0
      settings: SourceProductName=Simscape Electrical
  Trigonometric Function : Trigonometry
  rpm2Hz : Gain  Gain=15/60
  A : PMIOPort  Side=Right
  B : PMIOPort  Port=2  Side=Right
  C : PMIOPort  Port=3  Side=Right
  tag scope: Vabc_ref=global, input_freq=global
  wires:
  rpm2Hz/1 -> Hz2rad/s/1, [input_freq]
  Demux/3 -> Controlled Voltage Source2/1
  Demux/2 -> Controlled Voltage Source1/1
  Demux/1 -> Controlled Voltage Source/1
  Product/1 -> Demux/1, [Vabc_ref]
  Trigonometric Function/1 -> Product/2
  Sum/1 -> Trigonometric Function/1
  Hz2rad/s/1 -> Discrete-Time Integrator/1
  Constant/1 -> Sum/1
  Constant1/1 -> Product/1
  Discrete-Time Integrator/1 -> Sum/2
  rpm/1 -> rpm2Hz/1
  connections:
  Parasitic Resistive Load/LConn1 -- A/RConn1 -- Three-Phase V-I Measurement4/RConn1
  Parasitic Resistive Load/LConn2 -- B/RConn1 -- Three-Phase V-I Measurement4/RConn2
  Three-Phase V-I Measurement4/RConn3 -- Parasitic Resistive Load/LConn3 -- C/RConn1
  Three-Phase V-I Measurement4/LConn3 -- Controlled Voltage Source2/RConn1
  Three-Phase V-I Measurement4/LConn1 -- Controlled Voltage Source/RConn1
  Three-Phase V-I Measurement4/LConn2 -- Controlled Voltage Source1/RConn1
  Controlled Voltage Source1/LConn1 -- Controlled Voltage Source2/LConn1 -- Ground2/LConn1 -- Controlled Voltage Source/LConn1

== system Generator_Lib/Generator/VSCF Cycloconverter/AC Generator Cycloconverter/Phase A Cycloconverter ==
  negative cycle : powerlib/Power Electronics/Universal Bridge  Arms=3  SnubberResistance=1e3  SnubberCapacitance=1e-7  Device=Thyristors  Ron=1e-5  Lon=0  ForwardVoltages="[  0  0  ]"  ForwardVoltage=0  GTOparameters=[ 10e-6 , 20e-6 ]  IGBTparameters=[ 1e-6 , 2e-6 ]  Measurements=None  Measurements_2=None  converterType=Rectifier
      settings: SourceProductName=Simscape Electrical
  positive cycle : powerlib/Power Electronics/Universal Bridge  Arms=3  SnubberResistance=1e3  SnubberCapacitance=1e-7  Device=Thyristors  Ron=1e-5  Lon=0  ForwardVoltages="[  0  0  ]"  ForwardVoltage=0  GTOparameters=[ 10e-6 , 20e-6 ]  IGBTparameters=[ 1e-6 , 2e-6 ]  Measurements=None  Measurements_2=None  converterType=Rectifier
      settings: SourceProductName=Simscape Electrical
  VA+ : PMIOPort  Tag=PMCPort  Side=Right
  VA- : PMIOPort  Tag=PMCPort  Port=2  Side=Right
  A : PMIOPort  Tag=PMCPort  Port=3  Side=Left
  B : PMIOPort  Tag=PMCPort  Port=4  Side=Left
  C : PMIOPort  Tag=PMCPort  Port=5  Side=Left
  wires:
  [PhAgn] -> negative cycle/1
  [PhAgp] -> positive cycle/1
  connections:
  negative cycle/RConn2 -- VA+/RConn1 -- positive cycle/RConn1
  VA-/RConn1 -- positive cycle/RConn2 -- negative cycle/RConn1
  negative cycle/LConn3 -- positive cycle/LConn3 -- C/RConn1
  negative cycle/LConn2 -- positive cycle/LConn2 -- B/RConn1
  negative cycle/LConn1 -- positive cycle/LConn1 -- A/RConn1

== system Generator_Lib/Generator/VSCF Cycloconverter/AC Generator Cycloconverter/Phase B Cycloconverter ==
  negative cycle : powerlib/Power Electronics/Universal Bridge  Arms=3  SnubberResistance=1e3  SnubberCapacitance=1e-7  Device=Thyristors  Ron=1e-5  Lon=0  ForwardVoltages="[  0  0  ]"  ForwardVoltage=0  GTOparameters=[ 10e-6 , 20e-6 ]  IGBTparameters=[ 1e-6 , 2e-6 ]  Measurements=None  Measurements_2=None  converterType=Rectifier
      settings: SourceProductName=Simscape Electrical
  positive cycle : powerlib/Power Electronics/Universal Bridge  Arms=3  SnubberResistance=1e3  SnubberCapacitance=1e-7  Device=Thyristors  Ron=1e-5  Lon=0  ForwardVoltages="[  0  0  ]"  ForwardVoltage=0  GTOparameters=[ 10e-6 , 20e-6 ]  IGBTparameters=[ 1e-6 , 2e-6 ]  Measurements=None  Measurements_2=None  converterType=Rectifier
      settings: SourceProductName=Simscape Electrical
  VB+ : PMIOPort  Tag=PMCPort  Side=Right
  VB- : PMIOPort  Tag=PMCPort  Port=2  Side=Right
  A : PMIOPort  Tag=PMCPort  Port=3  Side=Left
  B : PMIOPort  Tag=PMCPort  Port=4  Side=Left
  C : PMIOPort  Tag=PMCPort  Port=5  Side=Left
  wires:
  [PhBgp] -> positive cycle/1
  [PhBgn] -> negative cycle/1
  connections:
  A/RConn1 -- positive cycle/LConn1 -- negative cycle/LConn1
  positive cycle/LConn2 -- B/RConn1 -- negative cycle/LConn2
  C/RConn1 -- positive cycle/LConn3 -- negative cycle/LConn3
  negative cycle/RConn1 -- positive cycle/RConn2 -- VB-/RConn1
  positive cycle/RConn1 -- VB+/RConn1 -- negative cycle/RConn2

== system Generator_Lib/Generator/VSCF Cycloconverter/AC Generator Cycloconverter/Phase C Cycloconverter ==
  negative cycle : powerlib/Power Electronics/Universal Bridge  Arms=3  SnubberResistance=1e3  SnubberCapacitance=1e-7  Device=Thyristors  Ron=1e-5  Lon=0  ForwardVoltages="[  0  0  ]"  ForwardVoltage=0  GTOparameters=[ 10e-6 , 20e-6 ]  IGBTparameters=[ 1e-6 , 2e-6 ]  Measurements=None  Measurements_2=None  converterType=Rectifier
      settings: SourceProductName=Simscape Electrical
  positive cycle : powerlib/Power Electronics/Universal Bridge  Arms=3  SnubberResistance=1e3  SnubberCapacitance=1e-7  Device=Thyristors  Ron=1e-5  Lon=0  ForwardVoltages="[  0  0  ]"  ForwardVoltage=0  GTOparameters=[ 10e-6 , 20e-6 ]  IGBTparameters=[ 1e-6 , 2e-6 ]  Measurements=None  Measurements_2=None  converterType=Rectifier
      settings: SourceProductName=Simscape Electrical
  VC+ : PMIOPort  Tag=PMCPort  Side=Right
  VC- : PMIOPort  Tag=PMCPort  Port=2  Side=Right
  A : PMIOPort  Tag=PMCPort  Port=3  Side=Left
  B : PMIOPort  Tag=PMCPort  Port=4  Side=Left
  C : PMIOPort  Tag=PMCPort  Port=5  Side=Left
  wires:
  [PhCgn] -> negative cycle/1
  [PhCgp] -> positive cycle/1
  connections:
  negative cycle/RConn2 -- VC+/RConn1 -- positive cycle/RConn1
  VC-/RConn1 -- positive cycle/RConn2 -- negative cycle/RConn1
  negative cycle/LConn3 -- positive cycle/LConn3 -- C/RConn1
  negative cycle/LConn2 -- positive cycle/LConn2 -- B/RConn1
  negative cycle/LConn1 -- positive cycle/LConn1 -- A/RConn1

== system Generator_Lib/Generator/VSCF Cycloconverter/Generator Control Breaker (GCB)/Close switch ==
  In1 : Inport
  Data Type Conversion : DataTypeConversion
  Rad_Rpm : Gain  Gain=30/pi
  Relay : Relay  OnSwitchValue=9000  OffSwitchValue=8900
  Out1 : Outport
  wires:
  Data Type Conversion/1 -> Out1/1
  Rad_Rpm/1 -> Relay/1
  Relay/1 -> Data Type Conversion/1
  In1/1 -> Rad_Rpm/1

== system Generator_Lib/Generator/VSCF Cycloconverter/Generator Control Breaker (GCB)/Contactor ==
  com : Inport
  Three-Phase Breaker : powerlib/Elements/Three-Phase Breaker  InitialState=open  SwitchA=on  SwitchB=on  SwitchC=on  SwitchTimes="[4/60  10/60]"  External=on  BreakerResistance=0.001  SnubberResistance=1e3  SnubberCapacitance=inf  Measurements=None
      settings: SourceProductName=Simscape Electrical
  A : PMIOPort  Side=Left
  a : PMIOPort  Port=2  Side=Right
  B : PMIOPort  Port=3  Side=Left
  b : PMIOPort  Port=4  Side=Right
  C : PMIOPort  Port=5  Side=Left
  c : PMIOPort  Port=6  Side=Right
  wires:
  com/1 -> Three-Phase Breaker/1
  connections:
  a/RConn1 -- Three-Phase Breaker/RConn1
  Three-Phase Breaker/RConn2 -- b/RConn1
  c/RConn1 -- Three-Phase Breaker/RConn3
  A/RConn1 -- Three-Phase Breaker/LConn1
  B/RConn1 -- Three-Phase Breaker/LConn2
  C/RConn1 -- Three-Phase Breaker/LConn3

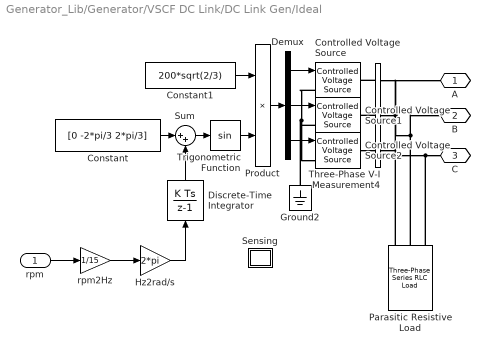
== system Generator_Lib/Generator/VSCF DC Link/DC Link Gen/Ideal ==
  rpm : Inport
  Constant : Constant  Value=[0 -2*pi/3 2*pi/3]
  Constant1 : Constant  Value=200*sqrt(2/3)
  Controlled Voltage Source : powerlib/Electrical Sources/Controlled Voltage Source  Initialize=off  Source_Type=AC  Amplitude=0  Phase=0  Frequency=0  Measurements=None
      settings: SourceProductName=Simscape Electrical
  Controlled Voltage Source1 : powerlib/Electrical Sources/Controlled Voltage Source  Initialize=off  Source_Type=AC  Amplitude=0  Phase=0  Frequency=0  Measurements=None
      settings: SourceProductName=Simscape Electrical
  Controlled Voltage Source2 : powerlib/Electrical Sources/Controlled Voltage Source  Initialize=off  Source_Type=AC  Amplitude=0  Phase=0  Frequency=0  Measurements=None
      settings: SourceProductName=Simscape Electrical
  Demux : Demux  Outputs=3
  Discrete-Time Integrator : DiscreteIntegrator  SampleTime=Ts  ICPrevOutput=DiscIntNeverNeededParam  ICPrevScaledInput=DiscIntNeverNeededParam
  Ground2 : powerlib/Elements/Ground  LConnTagsString=a
      settings: SourceProductName=Simscape Electrical
  Hz2rad/s : Gain  Gain=2*pi
  Parasitic Resistive Load : powerlib/Elements/Three-Phase Series RLC Load  LConnTagsString=A|B|C  Configuration=Y (grounded)  NominalVoltage=200  Vabc=[1e3 1e3 1e3]  Vabcp=[1e3 1e3 1e3]  NominalFrequency=400  UnbalancedPower=off  ActivePower=5000  InductivePower=0  CapacitivePower=0  Pabc=[10e3 9e3 11e3]  QLabc=[100 90 110]  QCabc=[100 90 110]  Pabcp=[10e3 9e3 11e3]  QLabcp=[100 90 110]  QCabcp=[100 90 110]  Measurements=None  LoadType=constant Z
      settings: SourceProductName=Simscape Electrical
  Product : Product
  Sensing : Subsystem
      mask Display: disp('S')
  Sum : Sum  Inputs=|++
  Three-Phase V-I Measurement4 : powerlib/Measurements/Three-Phase V-I Measurement  VoltageMeasurement=phase-to-ground  SetLabelV=on  LabelV=Vabc_Gen1Only  Vpu=off  VpuLL=off  CurrentMeasurement=yes  SetLabelI=on  LabelI=Iabc_Gen1Only  Ipu=off  Pbase=100e6  Vbase=500e3  OutputType=Magnitude  PhasorSimulation=on  PSBequivalent=0
      settings: SourceProductName=Simscape Electrical
  Trigonometric Function : Trigonometry
  rpm2Hz : Gain  Gain=1/15
  A : PMIOPort  Side=Right
  B : PMIOPort  Port=2  Side=Right
  C : PMIOPort  Port=3  Side=Right
  wires:
  rpm/1 -> rpm2Hz/1
  Discrete-Time Integrator/1 -> Sum/2
  Constant1/1 -> Product/1
  Constant/1 -> Sum/1
  Hz2rad/s/1 -> Discrete-Time Integrator/1
  Sum/1 -> Trigonometric Function/1
  Trigonometric Function/1 -> Product/2
  Product/1 -> Demux/1
  Demux/1 -> Controlled Voltage Source/1
  Demux/2 -> Controlled Voltage Source1/1
  Demux/3 -> Controlled Voltage Source2/1
  rpm2Hz/1 -> Hz2rad/s/1
  connections:
  Controlled Voltage Source/LConn1 -- Ground2/LConn1 -- Controlled Voltage Source2/LConn1 -- Controlled Voltage Source1/LConn1
  Three-Phase V-I Measurement4/LConn1 -- Controlled Voltage Source/RConn1
  Three-Phase V-I Measurement4/LConn2 -- Controlled Voltage Source1/RConn1
  Controlled Voltage Source2/RConn1 -- Three-Phase V-I Measurement4/LConn3
  Three-Phase V-I Measurement4/RConn3 -- Parasitic Resistive Load/LConn3 -- C/RConn1
  Three-Phase V-I Measurement4/RConn2 -- Parasitic Resistive Load/LConn2 -- B/RConn1
  Three-Phase V-I Measurement4/RConn1 -- A/RConn1 -- Parasitic Resistive Load/LConn1

== system Generator_Lib/Generator/VSCF DC Link/DC Link Gen/Sync Mach ==
  rpm : Inport
  Bus Selector2 : BusSelector  OutputSignals=Rotor speed wm (rad/s)
  Displays : Subsystem
  Generator Control Unit (GCU) : Subsystem
      mask Display: %image(imread('power_aircraft_distribution_GCU.jpg','jpg'))
  Generator Control Breaker (GCB) : Subsystem
  Parasitic Resistive Load1 : powerlib/Elements/Three-Phase Series RLC Load  LConnTagsString=A|B|C  Configuration=Y (grounded)  NominalVoltage=200  Vabc=[1e3 1e3 1e3]  Vabcp=[1e3 1e3 1e3]  NominalFrequency=800  UnbalancedPower=off  ActivePower=5000  InductivePower=0  CapacitivePower=0  Pabc=[10e3 9e3 11e3]  QLabc=[100 90 110]  QCabc=[100 90 110]  Pabcp=[10e3 9e3 11e3]  QLabcp=[100 90 110]  QCabcp=[100 90 110]  Measurements=None  LoadType=constant Z
      settings: SourceProductName=Simscape Electrical
  Sensing : Subsystem
      mask Display: disp('S')
  Simplified Synchronous Machine SI Units1 : powerlib/Machines/Simplified Synchronous Machine SI Units  ConnectionType=3-wire Y  MechanicalLoad=Speed w  MeasurementBus=on  NominalParameters=[50e3 200 800]  Mechanical=[0.02 0 2*2]  InternalRL="[0.0204  0.08104e-3]"  InitialConditions=[-99 1.73677 24.5109 24.5109 24.5109 -1.98949 -121.989 118.011]  Units=1  LoadFlowParameters=[1,0,0,0,0]  TsPowergui=0  TsBlock=-1  BusType=swing  Pref=0  Qref=0  Qmin=-inf  Qmax=+inf  PLF=0  QLF=0
      settings: SourceProductName=Simscape Electrical  SourceProductBaseCode=PS
  Vab : Subsystem
  rpm2 radps : Gain  Gain=pi/30
  A : PMIOPort  Side=Right
  B : PMIOPort  Port=2  Side=Right
  C : PMIOPort  Port=3  Side=Right
  wires:
  rpm/1 -> rpm2 radps/1
  Generator Control Breaker (GCB)/2(Iabc) -> Generator Control Unit (GCU)/1(Iabc)
  Generator Control Unit (GCU)/1(V Field) -> Simplified Synchronous Machine SI Units1/2  "Field"
  Bus Selector2/1 -> Generator Control Breaker (GCB)/1(GLC), Generator Control Unit (GCU)/3(PMG), Displays/1(w)  "<Rotor speed wm (rad/s)>"
  Generator Control Breaker (GCB)/1(Vabc) -> Generator Control Unit (GCU)/2(Vabc)
  rpm2 radps/1 -> Simplified Synchronous Machine SI Units1/1
  Simplified Synchronous Machine SI Units1/1 -> Sensing/1(In1), Bus Selector2/1
  connections:
  C/RConn1 -- Generator Control Breaker (GCB)/RConn3
  Simplified Synchronous Machine SI Units1/RConn1 -- Generator Control Breaker (GCB)/LConn1 -- Parasitic Resistive Load1/LConn1
  Generator Control Breaker (GCB)/LConn2 -- Parasitic Resistive Load1/LConn2 -- Simplified Synchronous Machine SI Units1/RConn2
  Generator Control Breaker (GCB)/LConn3 -- Parasitic Resistive Load1/LConn3 -- Simplified Synchronous Machine SI Units1/RConn3
  Generator Control Breaker (GCB)/RConn2 -- B/RConn1 -- Vab/RConn2
  Generator Control Breaker (GCB)/RConn1 -- A/RConn1 -- Vab/RConn1

== system Generator_Lib/Generator/VSCF DC Link/Rect and Inv/Subsystem3 ==
  Vdc : powerlib/Measurements/Voltage Measurement  Tag=PoWeRsYsTeMmEaSuReMeNt  PhasorSimulation=off  OutputType=Magnitude  PSBequivalent=0
      settings: SourceProductName=Simscape Electrical
  + : PMIOPort  Side=Left
  - : PMIOPort  Port=2  Side=Right
  tag scope: Vdc_GenDCLink=global
  wires:
  Vdc/1 -> [Vdc_GenDCLink]  "Vdc"
  connections:
  -/RConn1 -- Vdc/LConn2
  Vdc/LConn1 -- +/RConn1
